simulink model "fcn"  (R2019a)
settings: Solver=ode3  StartTime=0.0  StopTime=100  FixedStep=0.01  RelTol=1e-3
libraries: simulink x1
settings Model: Creator=ASUS  LastModifiedBy=ASUS
settings DataIOCC: ReturnWorkspaceOutputs=off

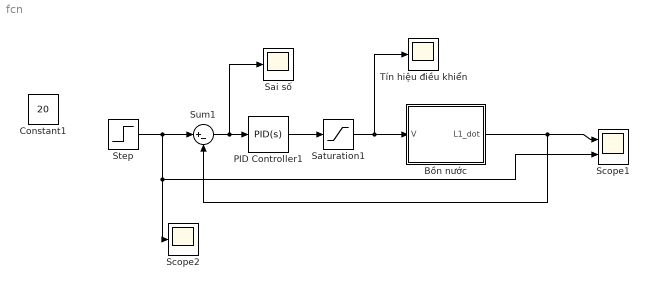
== system fcn ==
  Bồn nước : Subsystem
  Constant1 : Constant  Value=20
  PID Controller1 : simulink/Continuous/PID Controller  Controller=PID  Form=Parallel  TimeDomain=Continuous-time  SampleTime=-1  IntegratorMethod=Forward Euler  FilterMethod=Forward Euler  ControllerParametersSource=internal  P=20  I=0.01  D=0  UseFilter=on  N=100  TunerSelectOption=Transfer Function Based (PID Tuner App)  InitialConditionSource=internal  InitialConditionForIntegrator=0  InitialConditionForFilter=0  DifferentiatorICPrevScaledInput=0  ExternalReset=none  TrackingMode=off  Kt=1  LimitOutput=off  UpperSaturationLimit=inf  LowerSaturationLimit=-inf  LinearizeAsGain=on  AntiWindupMode=none  Kb=1  POutMin=[]  POutMax=[]  IOutMin=[]  IOutMax=[]  DOutMin=[]  DOutMax=[]  NOutMin=[]  NOutMax=[]  SumOutMin=[]  SumOutMax=[]  SaturationOutMin=[]  SaturationOutMax=[]  PParamMin=[]  PParamMax=[]  IParamMin=[]  IParamMax=[]  DParamMin=[]  DParamMax=[]  NParamMin=[]  NParamMax=[]  KbParamMin=[]  KbParamMax=[]  KtParamMin=[]  KtParamMax=[]  KbOutMin=[]  KbOutMax=[]  KtOutMin=[]  KtOutMax=[]  IntegratorOutMin=[]  IntegratorOutMax=[]  FilterOutMin=[]  FilterOutMax=[]  SumI1OutMin=[]  SumI1OutMax=[]  SumI2OutMin=[]  SumI2OutMax=[]  SumI3OutMin=[]  SumI3OutMax=[]  SumI4OutMin=[]  SumI4OutMax=[]  SumDOutMin=[]  SumDOutMax=[]  DifferentiatorOutMin=[]  DifferentiatorOutMax=[]  FilterDiffOutCoefMin=[]  FilterDiffOutCoefMax=[]  ReciprocalOutMin=[]  ReciprocalOutMax=[]  SumDenOutMin=[]  SumDenOutMax=[]  SumNumOutMin=[]  SumNumOutMax=[]  DivideOutMin=[]  DivideOutMax=[]  IntegratorContinuousStateAttributes=''  IntegratorStateMustResolveToSignalObject=off  IntegratorRTWStateStorageClass=Auto  FilterContinuousStateAttributes=''  FilterStateMustResolveToSignalObject=off  FilterRTWStateStorageClass=Auto  ParallelPVariant=InternalParameters  IdealPVariant=Disabled  IVariant=InternalParameters  DVariant=InternalParameters  IntegratorVariant=Continuous  SatVariant=Disabled  AWVariant=Passthrough  PCopyVariant=Disabled  TRVariant=Disabled  FdbkBlocksVariant=Forward  IdealPFdbkVariant=Disabled  SatFdbkVariant=Disabled  DerivativeFilterVariant=ContFilter  NVariant=InternalParameters  NCopyVariant=Disabled  FilterICVariant=InternalICsFilter  IntegratorICVariant=InternalICs  ExternalResetVariant=Disabled  TRSumVariant=Passthrough  SumFdbkVariant=Disabled  SumVariant=Sum_PID
  Sai số : Scope
  Saturation1 : Saturate  UpperLimit=22  LowerLimit=0
  Scope1 : Scope  NumInputPorts=2
  Scope2 : Scope
  Step : Step  Time=15  Before=15  After=25  SampleTime=0
  Sum1 : Sum  Inputs=|+-
  Tín hiệu điều khiển : Scope
  wires:
  Sum1/1 -> Sai số/1, PID Controller1/1
  PID Controller1/1 -> Saturation1/1
  Bồn nước/1(L1_dot) -> Scope1/1, Sum1/2
  Saturation1/1 -> Tín hiệu điều khiển/1, Bồn nước/1(V)
  Step/1 -> Scope1/2, Scope2/1, Sum1/1

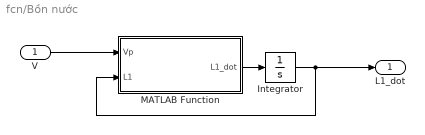
== system fcn/Bồn nước ==
  V : Inport
  Integrator : Integrator
  MATLAB Function : MATLAB Function  TreatAsAtomicUnit=on
  L1_dot : Outport
  wires:
  MATLAB Function/1(L1_dot) -> Integrator/1
  V/1 -> MATLAB Function/1(Vp)
  Integrator/1 -> L1_dot/1, MATLAB Function/2(L1)

== matlab function fcn/Bồn nước/MATLAB Function ==
  data: Vp input; L1 input; L1_dot output
function L1_dot= BON_NUOC(Vp,L1)
Km=4.6;
A1=15.5179;
a1=0.2;
g=9.8;
%equation
L1_dot=-(a1/A1)*sqrt(2*g*L1)+(Km/A1)*Vp;
